simulink model "sim_tcyb_2024_obs"  (R2020a)
settings: Solver=ode4  StartTime=0.0  StopTime=30.0  FixedStep=0.01  RelTol=1e-3
values from neighbouring files (symbols this model uses):
  k1 = 30    [init_tcyb_2024_obs.m]
  k2 = 30    [init_tcyb_2024_obs.m]
  kai_1_t = 0.02    [init_tcyb_2024_obs.m]
  kai_3_t = 0.1    [init_tcyb_2024_obs.m]
  l1 = 20    [init_tcyb_2024_obs.m]
  l2 = 20    [init_tcyb_2024_obs.m]
  Mii = diag([1;0;0;0;1])    [init_tcyb_2024_obs.m]
  pos0 = zeros(3, 1)    [init_tcyb_2024_obs.m]
  PZ0 = P0(3)    [init_tcyb_2024_obs.m]
  PZ1 = 10    [init_tcyb_2024_obs.m]
  R0 = 4    [init_tcyb_2024_obs.m]
  r1 = 20    [init_tcyb_2024_obs.m]
  R1 = 8    [init_tcyb_2024_obs.m]
  r2 = 20    [init_tcyb_2024_obs.m]
  Rx2 = 10    [init_tcyb_2024_obs.m]
  Ry2 = 6    [init_tcyb_2024_obs.m]
  Rz2 = 4    [init_tcyb_2024_obs.m]
  T0 = 0    [init_tcyb_2024_obs.m]
  T1 = tseq1    (= 10)    [init_tcyb_2024_obs.m]
  T12 = tseq1 + tseq12    (= 20)    [init_tcyb_2024_obs.m]
  T2 = tseq1 + tseq12 + tseq2    (= 30)    [init_tcyb_2024_obs.m]
  theta0 = ( 2 / 5 ) * pi    (= 1.25663706144)    [init_tcyb_2024_obs.m]
  vel0 = zeros(3, 1)    [init_tcyb_2024_obs.m]
  Wij = [0,0,1,0,0;              0,0,1,1,0;              1,0,0,0,1;              0,1,1,0,0;              0,0,1,0,0]    [init_tcyb_2024_obs.m]
  X1 = 8    [init_tcyb_2024_obs.m]
  X2 = 2    [init_tcyb_2024_obs.m]
  X3 = 3    [init_tcyb_2024_obs.m]
  Y1 = 10    [init_tcyb_2024_obs.m]
  Y2 = 2    [init_tcyb_2024_obs.m]
  Y3 = 4    [init_tcyb_2024_obs.m]
  Z1 = 4    [init_tcyb_2024_obs.m]
  Z2 = -6    [init_tcyb_2024_obs.m]
  Z3 = 2    [init_tcyb_2024_obs.m]
(part 2 of 2)

== matlab function sim_tcyb_2024_obs/cal lumped observation error agent 5 ==
  data: wij input; w0 input; ksi_d_est_vec input; ksi0 input; delta_ksi_vec input; eta_d_est_vec input; ksi_est_err_tilt_5 output; eta0 input; delta_eta_vec input; eta_est_err_tilt_5 output
function [ksi_est_err_tilt_5, eta_est_err_tilt_5]  = fcn(wij, w0, ksi_d_est_vec, ksi0, delta_ksi_vec, eta_d_est_vec, eta0, delta_eta_vec)
%%%% 计算跟随者期望速度分布式观测器误差
iiuav = 5;
ksi_est_err_tilt_5 = w0(iiuav, iiuav) * (ksi_d_est_vec(:,iiuav) - ksi0(:) - delta_ksi_vec(:,iiuav));
eta_est_err_tilt_5 = w0(iiuav, iiuav) * (eta_d_est_vec(:,iiuav) - eta0(:) - delta_eta_vec(:,iiuav));
for jjuav = 1:5
    ksi_est_err_tilt_5 = ksi_est_err_tilt_5 + ...
                                        wij(iiuav, jjuav) * ((ksi_d_est_vec(:,iiuav) - delta_ksi_vec(:,iiuav)) - (ksi_d_est_vec(:,jjuav) - delta_ksi_vec(:,jjuav)));
    eta_est_err_tilt_5 = eta_est_err_tilt_5 + ...
                                        wij(iiuav, jjuav) * ((eta_d_est_vec(:,iiuav) - delta_eta_vec(:,iiuav)) - (eta_d_est_vec(:,jjuav) - delta_eta_vec(:,jjuav)));
end

== matlab function sim_tcyb_2024_obs/cal position estimate error ==
  data: ksi_d_est_vec input; ksi_est_err output; ksi0 input; delta_ksi_vec input
function ksi_est_err  = fcn(ksi_d_est_vec, ksi0, delta_ksi_vec)
%%%% 计算跟随者期望位置分布式观测器误差
ksi_est_err = ksi_d_est_vec - repmat(ksi0, 1, 5) - delta_ksi_vec;

== matlab function sim_tcyb_2024_obs/cal velocity estimate error ==
  data: eta_d_est_vec input; eta_est_err output; eta0 input; delta_eta_vec input
function eta_est_err  = fcn(eta_d_est_vec, eta0, delta_eta_vec)
%%%% 计算跟随者期望速度分布式观测器误差
eta_est_err = eta_d_est_vec - repmat(eta0, 1, 5) - delta_eta_vec;

== matlab function sim_tcyb_2024_obs/combine follower desire velocity estimaters ==
  data: eta_d_est_1 input; eta_d_est_vec output; eta_d_est_2 input; eta_d_est_3 input; eta_d_est_4 input; eta_d_est_5 input
function eta_d_est_vec = fcn(eta_d_est_1, eta_d_est_2, eta_d_est_3, eta_d_est_4, eta_d_est_5)
%%%% 合并领导者位置观测器输出结果
eta_d_est_vec = [eta_d_est_1(:), eta_d_est_2(:), eta_d_est_3(:), eta_d_est_4(:), eta_d_est_5(:)];

== matlab function sim_tcyb_2024_obs/adaptive law c2i agent 1 ==
  data: r2 input; d_c2i_1 output; c2i_vec input; eta_est_err_tilt_vec input
function d_c2i_1 = fcn(r2, c2i_vec, eta_est_err_tilt_vec)
%%%% 自适应律 c2i
iiuav = 1;
d_c2i_1 = ( eta_est_err_tilt_vec(:,iiuav)' ) * eta_est_err_tilt_vec(:,iiuav) ...
                    - r2 * c2i_vec(iiuav);

== matlab function sim_tcyb_2024_obs/combine leader position estimaters ==
  data: ksi_d_est_1 input; ksi_d_est_vec output; ksi_d_est_2 input; ksi_d_est_3 input; ksi_d_est_4 input; ksi_d_est_5 input
function ksi_d_est_vec  = fcn(ksi_d_est_1, ksi_d_est_2, ksi_d_est_3, ksi_d_est_4, ksi_d_est_5)
%%%% 合并领导者位置观测器输出结果
ksi_d_est_vec = [ksi_d_est_1(:), ksi_d_est_2(:), ksi_d_est_3(:), ksi_d_est_4(:), ksi_d_est_5(:)];

== matlab function sim_tcyb_2024_obs/combine lumped follower observation error  ==
  data: ksi_est_err_tilt_1 input; ksi_est_err_tilt_2 input; ksi_est_err_tilt_3 input; ksi_est_err_tilt_4 input; ksi_est_err_tilt_5 input; ksi_est_err_tilt_vec output; eta_est_err_tilt_1 input; eta_est_err_tilt_vec output; eta_est_err_tilt_2 input; eta_est_err_tilt_3 input; eta_est_err_tilt_4 input; eta_est_err_tilt_5 input
function [ksi_est_err_tilt_vec, eta_est_err_tilt_vec]  = fcn(ksi_est_err_tilt_1, ksi_est_err_tilt_2, ksi_est_err_tilt_3, ksi_est_err_tilt_4, ksi_est_err_tilt_5, ...
                                                                                                        eta_est_err_tilt_1, eta_est_err_tilt_2, eta_est_err_tilt_3, eta_est_err_tilt_4, eta_est_err_tilt_5)
%%%% 合并领导者位置观测器输出结果
ksi_est_err_tilt_vec = [ksi_est_err_tilt_1, ksi_est_err_tilt_2, ksi_est_err_tilt_3, ksi_est_err_tilt_4, ksi_est_err_tilt_5];
eta_est_err_tilt_vec = [eta_est_err_tilt_1, eta_est_err_tilt_2, eta_est_err_tilt_3, eta_est_err_tilt_4, eta_est_err_tilt_5];

== matlab function sim_tcyb_2024_obs/divide eta_est_err ==
  data: eta_est_err input; eta_est_err_1 output; eta_est_err_2 output; eta_est_err_3 output; eta_est_err_4 output; eta_est_err_5 output
function [eta_est_err_1, eta_est_err_2, eta_est_err_3, eta_est_err_4, eta_est_err_5]  = fcn(eta_est_err)
%%%% 计算跟随者期望位置分布式观测器误差
eta_est_err_1 = eta_est_err(:,1);
eta_est_err_2 = eta_est_err(:,2);
eta_est_err_3 = eta_est_err(:,3);
eta_est_err_4 = eta_est_err(:,4);
eta_est_err_5 = eta_est_err(:,5);

== matlab function sim_tcyb_2024_obs/divide ksi_est_err ==
  data: ksi_est_err input; ksi_est_err_1 output; ksi_est_err_2 output; ksi_est_err_3 output; ksi_est_err_4 output; ksi_est_err_5 output
function [ksi_est_err_1, ksi_est_err_2, ksi_est_err_3, ksi_est_err_4, ksi_est_err_5]  = fcn(ksi_est_err)
%%%% 计算跟随者期望位置分布式观测器误差
ksi_est_err_1 = ksi_est_err(:,1);
ksi_est_err_2 = ksi_est_err(:,2);
ksi_est_err_3 = ksi_est_err(:,3);
ksi_est_err_4 = ksi_est_err(:,4);
ksi_est_err_5 = ksi_est_err(:,5);

== matlab function sim_tcyb_2024_obs/distributed follower desire velocity observer agent 1 ==
  data: k2 input; d_eta_d_est_1 output; l2 input; c2i_vec input; u0 input; eta_est_err_tilt_vec input
function d_eta_d_est_1 = fcn(k2, l2, c2i_vec, u0, eta_est_err_tilt_vec)
%%%% 跟随者期望速度分布式观测器
iiuav = 1;
d_eta_d_est_1 = u0(:) - ( c2i_vec(iiuav) ^ 2 ) * eta_est_err_tilt_vec(:,iiuav) ...
                                - k2 * eta_est_err_tilt_vec(:,iiuav) ...
                                - l2 * sign( eta_est_err_tilt_vec(:,iiuav) );

== matlab function sim_tcyb_2024_obs/adaptive law c2i agent 2 ==
  data: r2 input; d_c2i_2 output; c2i_vec input; eta_est_err_tilt_vec input
function d_c2i_2 = fcn(r2, c2i_vec, eta_est_err_tilt_vec)
%%%% 自适应律 c2i
iiuav = 2;
d_c2i_2 = ( eta_est_err_tilt_vec(:,iiuav)' ) * eta_est_err_tilt_vec(:,iiuav) ...
                    - r2 * c2i_vec(iiuav);

== matlab function sim_tcyb_2024_obs/adaptive law c2i agent 3 ==
  data: r2 input; d_c2i_3 output; c2i_vec input; eta_est_err_tilt_vec input
function d_c2i_3 = fcn(r2, c2i_vec, eta_est_err_tilt_vec)
%%%% 自适应律 c2i
iiuav = 3;
d_c2i_3 = ( eta_est_err_tilt_vec(:,iiuav)' ) * eta_est_err_tilt_vec(:,iiuav) ...
                    - r2 * c2i_vec(iiuav);

== matlab function sim_tcyb_2024_obs/adaptive law c2i agent 4 ==
  data: r2 input; d_c2i_4 output; c2i_vec input; eta_est_err_tilt_vec input
function d_c2i_4 = fcn(r2, c2i_vec, eta_est_err_tilt_vec)
%%%% 自适应律 c2i
iiuav = 4;
d_c2i_4 = ( eta_est_err_tilt_vec(:,iiuav)' ) * eta_est_err_tilt_vec(:,iiuav) ...
                    - r2 * c2i_vec(iiuav);

== matlab function sim_tcyb_2024_obs/adaptive law c2i agent 5 ==
  data: r2 input; d_c2i_5 output; c2i_vec input; eta_est_err_tilt_vec input
function d_c2i_5 = fcn(r2, c2i_vec, eta_est_err_tilt_vec)
%%%% 自适应律 c2i
iiuav = 5;
d_c2i_5 = ( eta_est_err_tilt_vec(:,iiuav)' ) * eta_est_err_tilt_vec(:,iiuav) ...
                    - r2 * c2i_vec(iiuav);

== matlab function sim_tcyb_2024_obs/combine c2i ==
  data: c2i_1 input; c2i_vec output; c2i_2 input; c2i_3 input; c2i_4 input; c2i_5 input
function c2i_vec = fcn(c2i_1, c2i_2, c2i_3, c2i_4, c2i_5)
%%%% 合并自适应律
c2i_vec = [c2i_1, c2i_2, c2i_3, c2i_4, c2i_5];

== matlab function sim_tcyb_2024_obs/adaptive law c1i agent 2 ==
  data: r1 input; d_c1i_2 output; c1i_vec input; ksi_est_err_tilt_vec input
function d_c1i_2 = fcn(r1, c1i_vec, ksi_est_err_tilt_vec)
%%%% 自适应律 c1i
iiuav = 2;
d_c1i_2 = ( ksi_est_err_tilt_vec(:,iiuav)' ) * ksi_est_err_tilt_vec(:,iiuav) ...
                    - r1 * c1i_vec(iiuav);
